simulink model "determine_attitude_quest"  (R2022a)
settings: Solver=VariableStepAuto  StartTime=0.0  StopTime=10.0  RelTol=1e-3
undefined symbols (not defined in the file or in its folder): IAU, km, s
libraries: aerolibutil x9, sharedtransform x3, vrlib x3, aerolibtransform2 x2, aerolibcelestial x1
settings Model: Creator=joshu  LastModifiedBy=joshu

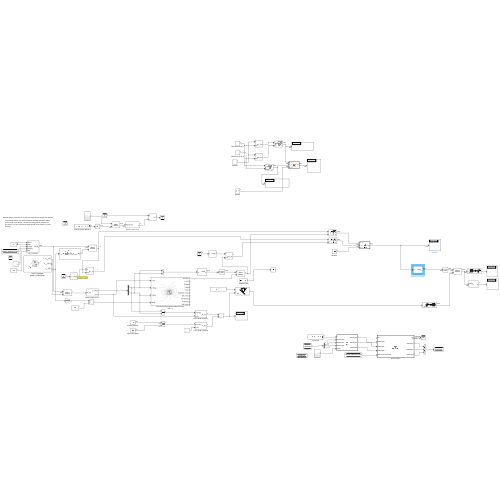
[thumbnail: Simulink's stored preview of the top-level diagram]
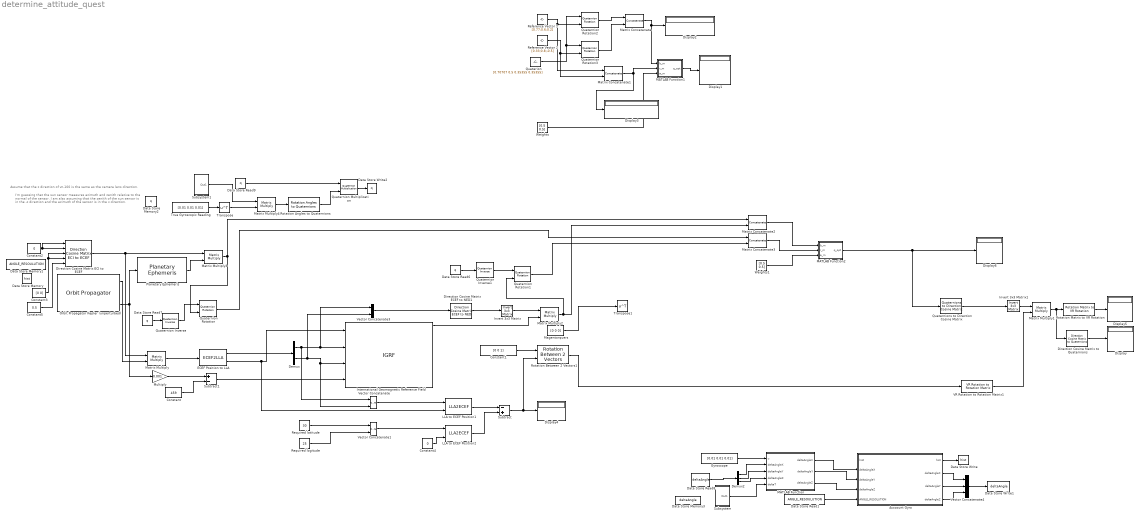
== system determine_attitude_quest ==
  note: I'm guessing that the sun sensor measures azimuth and zenith relative to the normal of the sensor. I am also assuming that the zenith of the sun sensor is in the -z direction and the azimuth of the sensor is in the x direction.
  note: Assume that the z direction of vn-100 is the same as the camera lens direction.
  Acccount Gyro : MATLAB Function  TreatAsAtomicUnit=on
  Constant : Constant  Value=459
  Constant1 : Constant  Value=[0 0 1]
  Constant2 : Constant  Value=0
  Constant3 : Constant  Value=[0 0]
  Constant4 : Constant  Value=0
  Constant5 : Constant  Value=0.5
  Data Store Memory : DataStoreMemory  DataStoreName=hist  WriteAfterWriteMsg=warning  InitialValue=1  ShowAdditionalParam=off  OutDataTypeStr=double  Dimensions=[100 100 100]
  Data Store Memory1 : DataStoreMemory  DataStoreName=ANGLE_RESOULUTION  WriteAfterWriteMsg=warning  InitialValue=100  ShowAdditionalParam=off
  Data Store Memory2 : DataStoreMemory  DataStoreName=q  WriteAfterWriteMsg=warning  InitialValue=[0.70707 0.5 0.35355 0.35355]  ShowAdditionalParam=off
  Data Store Memory3 : DataStoreMemory  DataStoreName=deltaAngle  WriteAfterWriteMsg=warning  InitialValue=[0 0 0]  ShowAdditionalParam=off
  Data Store Read1 : DataStoreRead  DataStoreName=ANGLE_RESOULUTION  IndexOptions=Index vector (dialog)  Indices=1  OutputSizes=1
  Data Store Read6 : DataStoreRead  DataStoreName=q  IndexOptions=Index vector (dialog)  Indices=1  OutputSizes=1
  Data Store Read7 : DataStoreRead  DataStoreName=q  IndexOptions=Index vector (dialog)  Indices=1  OutputSizes=1
  Data Store Read8 : DataStoreRead  DataStoreName=deltaAngle  IndexOptions=Index vector (dialog)  Indices=1  OutputSizes=1
  Data Store Read9 : DataStoreRead  DataStoreName=q  IndexOptions=Index vector (dialog)  Indices=1  OutputSizes=1
  Data Store Write : DataStoreWrite  DataStoreName=hist  IndexOptions=Index vector (dialog)  Indices=1  OutputSizes=1
  Data Store Write1 : DataStoreWrite  DataStoreName=deltaAngle  IndexOptions=Index vector (dialog)  Indices=1  OutputSizes=1
  Data Store Write2 : DataStoreWrite  DataStoreName=q  IndexOptions=Index vector (dialog)  Indices=1  OutputSizes=1
  Demux : Demux  Outputs=2
  Demux2 : Demux  Outputs=3
  Direction Cosine Matrix ECEF to NED1 : aerolibtransform2/Direction Cosine Matrix ECEF to NED
      settings: SourceProductBaseCode=AE
  Direction Cosine Matrix ECI to ECEF : aerolibtransform2/Direction Cosine Matrix ECI to ECEF  red=IAU-2000/2006  year=2013  month=January  day=1  hour=0  min=0  sec=0  deltaT=Day  errorflag=Error  extraparamflag=on
      settings: AttributesFormatString=%<red>  SourceProductBaseCode=AE
  Direction Cosine Matrix to Quaternions : sharedtransform/Direction Cosine Matrix  to Quaternions  aMode=0  action=None  tolerance=eps(2)
      settings: SourceProductBaseCode=AE,PW,DR,MT,VE
  Display{,1..6} (7 alike) : Display
  ECEF Position to LLA : ECEF2LLA
  Gyroscope : Constant  Value=[0.01 0.01 0.01]
  International Geomagnetic Reference Field : IGRF  month=January  day=1  year=2020  action=Warning
      settings: AttributesFormatString=%<generation>
  Invert 3x3 Matrix : aerolibutil/Invert  3x3 Matrix
  Invert 3x3 Matrix1 : aerolibutil/Invert  3x3 Matrix
  LLA to ECEF Position1 : LLA2ECEF
  LLA to ECEF Position2 : LLA2ECEF
  MATLAB Function : MATLAB Function  TreatAsAtomicUnit=on
  MATLAB Function1 : MATLAB Function  TreatAsAtomicUnit=on
  MATLAB Function2 : MATLAB Function  TreatAsAtomicUnit=on
  Magentorquers : Constant  Value=[0 0 0]
  Matrix Concatenate{,1..3} (4 alike) : Concatenate  Mode=Multidimensional array  ConcatenateDimension=2
  Matrix Multiply{,1..4} (5 alike) : Product  Multiplication=Matrix(*)
  Multiply : Gain  Gain=0.001
  Orbit Propagator Kepler (unperturbed) : OrbitPropagator  inertialPosition=[3649700.0 3308200.0 -4676600.0]  inertialVelocity=[-2750.8 6666.4 2573.4]  fixedPosition=[-4142689.0 -2676864.7 -4669861.6]  fixedVelocity=[1452.7 -6720.7 2568.1]  customR=3396200  customMu=4.305e13  customJ2=1.0826269e-03  customOmega=4.06125949e-3
  Planetary Ephemeris : aerolibcelestial/Planetary Ephemeris  kmflag=km,km/s  epochflag=Julian date  de=DE405  nCenter=Earth  nTarget=Sun  errorflag=Error  velflag=off
      settings: SourceProductBaseCode=AE
  Quaterion : Constant  Value=[0.70707 0.5 0.35355 0.35355]
  Quaternion Inverse : aerolibutil/Quaternion Inverse
  Quaternion Inverse1 : aerolibutil/Quaternion Inverse
  Quaternion Multiplication : aerolibutil/Quaternion Multiplication
  Quaternion Rotation{,1..3} (4 alike) : aerolibutil/Quaternion Rotation
  Quaternions to Direction Cosine Matrix : sharedtransform/Quaternions to  Direction Cosine Matrix  aMode=aMode
      settings: SourceProductBaseCode=AE,PW,DR,MT,VE
  Reference Vector 1 : Constant  Value=[0.77;0.6;0.2]
  Reference Vector 2 : Constant  Value=[0.33;0.8;-0.5]
  Required latitude : Constant  Value=30  VectorParams1D=off
  Required logitude : Constant  Value=25  VectorParams1D=off
  Rotation Angles to Quaternions : sharedtransform/Rotation Angles to Quaternions  rotationOrder=ZYX  aMode=aMode
      settings: SourceProductBaseCode=AE,PW,DR,MT,VE
  Rotation Between 2 Vectors1 : vrlib/Utilities/Rotation Between 2 Vectors
      settings: SourceProductBaseCode=SL
  Rotation Matrix to VR Rotation : vrlib/Utilities/Rotation Matrix to VR Rotation  maxzero=1e-12
      settings: SourceProductBaseCode=SL
  Subsystem : Subsystem
  Subsystem1 : Subsystem
  Subtract : Sum  Inputs=-+
  Subtract1 : Sum  Inputs=+-
  Transpose : Math  Operator=transpose
  Transpose1 : Math  Operator=transpose
  True Gyroscopic Reading : Constant  Value=[0.01 0.01 0.01]
  VR Rotation to Rotation Matrix1 : vrlib/Utilities/VR Rotation to Rotation Matrix  maxzero=1e-12
      settings: SourceProductBaseCode=SL
  Vector Concatenate : Concatenate
  Vector Concatenate1 : Concatenate
  Vector Concatenate3 : Concatenate
  Vector Concatenate4 : Concatenate  NumInputs=3
  Weights : Constant  Value=[0.5 0.5]
  Weights1 : Constant  Value=[0.5 0.5]
  wires:
  Quaternion Rotation1/1 -> Matrix Concatenate3/2
  Rotation Between 2 Vectors1/1 -> VR Rotation to Rotation Matrix1/1
  Subtract/1 -> Rotation Between 2 Vectors1/2, Display4/1
  MATLAB Function2/1(q_opt) -> Quaternions to Direction Cosine Matrix/1, Display6/1
  Data Store Read1/1 -> Acccount Gyro/5(ANGLE_RESOLUTION)
  Invert 3x3 Matrix1/1 -> Matrix Multiply1/1
  Direction Cosine Matrix ECEF to NED1/1 -> Invert 3x3 Matrix/1
  Acccount Gyro/1(hist) -> Data Store Write/1
  Subtract1/1 -> International Geomagnetic Reference Field/4
  Gyroscope/1 -> MATLAB Function/1(u)
  VR Rotation to Rotation Matrix1/1 -> Matrix Multiply1/2
  Vector Concatenate1/1 -> LLA to ECEF Position2/1
  Rotation Matrix to VR Rotation/1 -> Display5/1
  Vector Concatenate3/1 -> Direction Cosine Matrix ECEF to NED1/1
  Constant5/1 -> Direction Cosine Matrix ECI to ECEF/5
  Orbit Propagator Kepler (unperturbed)/1 -> Matrix Multiply/2
  Constant4/1 -> LLA to ECEF Position2/2
  Matrix Multiply2/1 -> Matrix Concatenate2/2, Quaternion Rotation1/2
  ECEF Position to LLA/1 -> Demux/1
  Constant2/1 -> Direction Cosine Matrix ECI to ECEF/2, Direction Cosine Matrix ECI to ECEF/1
  Direction Cosine Matrix to Quaternions/1 -> Display/1
  ECEF Position to LLA/2 -> LLA to ECEF Position1/2, International Geomagnetic Reference Field/1
  International Geomagnetic Reference Field/1 -> Matrix Multiply2/2
  Invert 3x3 Matrix/1 -> Matrix Multiply2/1
  Magentorquers/1 -> Transpose1/1
  LLA to ECEF Position1/1 -> Subtract/1
  Required logitude/1 -> Vector Concatenate1/2
  Direction Cosine Matrix ECI to ECEF/1 -> Matrix Multiply/1, Matrix Multiply3/1
  Required latitude/1 -> Vector Concatenate1/1
  Demux/2 -> Vector Concatenate/2, International Geomagnetic Reference Field/3, Vector Concatenate3/2
  Matrix Multiply/1 -> ECEF Position to LLA/1
  Matrix Multiply3/1 -> Matrix Concatenate2/1, Quaternion Rotation/2
  Planetary Ephemeris/1 -> Matrix Multiply3/2
  LLA to ECEF Position2/1 -> Subtract/2
  Vector Concatenate/1 -> LLA to ECEF Position1/1
  Multiply/1 -> Subtract1/1
  Quaternion Rotation/1 -> Matrix Concatenate3/1
  Constant1/1 -> Rotation Between 2 Vectors1/1
  Constant/1 -> Subtract1/2
  Demux/1 -> Vector Concatenate3/1, International Geomagnetic Reference Field/2, Vector Concatenate/1
  Matrix Multiply1/1 -> Rotation Matrix to VR Rotation/1, Direction Cosine Matrix to Quaternions/1
  Constant3/1 -> Direction Cosine Matrix ECI to ECEF/4, Direction Cosine Matrix ECI to ECEF/3
  Orbit Propagator Kepler (unperturbed)/3 -> Multiply/1, Planetary Ephemeris/1
  Quaternion Inverse/1 -> Quaternion Rotation/1
  Quaternion Inverse1/1 -> Quaternion Rotation1/1
  Data Store Read6/1 -> Quaternion Inverse1/1
  Data Store Read7/1 -> Quaternion Inverse/1
  Demux2/1 -> MATLAB Function/2("deltaAngleX ")
  Demux2/2 -> MATLAB Function/3("deltaAngleY ")
  Demux2/3 -> MATLAB Function/4("deltaAngleZ ")
  Subsystem/1(Out1) -> MATLAB Function/5(deltaT)
  MATLAB Function/1(deltaAngleX) -> Acccount Gyro/2("deltaAngleX ")
  MATLAB Function/2(deltaAngleY) -> Acccount Gyro/3("deltaAngleY ")
  MATLAB Function/3(deltaAngleZ) -> Acccount Gyro/4("deltaAngleZ ")
  Data Store Read8/1 -> Demux2/1
  Acccount Gyro/2(deltaAngleX) -> Vector Concatenate4/1
  Acccount Gyro/3(deltaAngleY) -> Vector Concatenate4/2
  Acccount Gyro/4(deltaAngleZ) -> Vector Concatenate4/3
  Vector Concatenate4/1 -> Data Store Write1/1
  True Gyroscopic Reading/1 -> Transpose/1
  Subsystem1/1(Out1) -> Matrix Multiply4/1
  Matrix Multiply4/1 -> Rotation Angles to Quaternions/1
  Data Store Read9/1 -> Quaternion Multiplication/1
  Rotation Angles to Quaternions/1 -> Quaternion Multiplication/2
  Quaternion Multiplication/1 -> Data Store Write2/1
  Transpose/1 -> Matrix Multiply4/2
  MATLAB Function1/1(q_opt) -> Display1/1
  Quaterion/1 -> Quaternion Rotation3/1, Quaternion Rotation2/1
  Reference Vector 2/1 -> Matrix Concatenate1/2, Quaternion Rotation3/2
  Reference Vector 1/1 -> Matrix Concatenate1/1, Quaternion Rotation2/2
  Quaternion Rotation2/1 -> Matrix Concatenate/1
  Quaternion Rotation3/1 -> Matrix Concatenate/2
  Weights/1 -> MATLAB Function1/3(a_m)
  Matrix Concatenate1/1 -> Display3/1, MATLAB Function1/2(r_m)
  Matrix Concatenate/1 -> Display2/1, MATLAB Function1/1(b_m)
  Matrix Concatenate2/1 -> MATLAB Function2/1(b_m)
  Matrix Concatenate3/1 -> MATLAB Function2/2(r_m)
  Weights1/1 -> MATLAB Function2/3(a_m)
  Quaternions to Direction Cosine Matrix/1 -> Invert 3x3 Matrix1/1

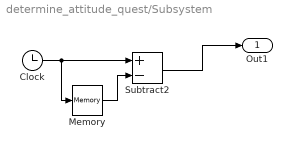
== system determine_attitude_quest/Subsystem ==
  Clock : Clock
  Memory : Memory
  Subtract2 : Sum  Inputs=+-
  Out1 : Outport
  wires:
  Memory/1 -> Subtract2/2
  Clock/1 -> Memory/1, Subtract2/1
  Subtract2/1 -> Out1/1

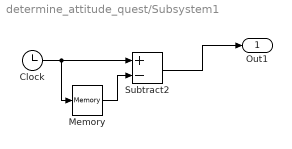
== system determine_attitude_quest/Subsystem1 ==
  Clock : Clock
  Memory : Memory
  Subtract2 : Sum  Inputs=+-
  Out1 : Outport
  wires:
  Memory/1 -> Subtract2/2
  Clock/1 -> Memory/1, Subtract2/1
  Subtract2/1 -> Out1/1

== matlab function determine_attitude_quest/Acccount Gyro ==
  data: hist input size=[100 100 100]; hist output; deltaAngleX input; deltaAngleY input; deltaAngleZ input; ANGLE_RESOLUTION input; deltaAngleX output; deltaAngleY output; deltaAngleZ output
function [hist,deltaAngleX,deltaAngleY,deltaAngleZ] = addMotion(hist,deltaAngleX,deltaAngleY,deltaAngleZ,ANGLE_RESOLUTION)
    %ANGLE_RESOLUTION = 500;

    if(deltaAngleX > 2*pi/ANGLE_RESOLUTION)
        hist = circshift(hist,1,1);
        deltaAngleX = deltaAngleX - 2*pi/ANGLE_RESOLUTION;
    end
    
    if(deltaAngleY > 2*pi/ANGLE_RESOLUTION)
        hist = circshift(hist,1,2);
        deltaAngleY = deltaAngleY - 2*pi/ANGLE_RESOLUTION;
    end
    
    if(deltaAngleZ > 2*pi/ANGLE_RESOLUTION)
        hist = circshift(hist,1,3);
        deltaAngleZ = deltaAngleZ - 2*pi/ANGLE_RESOLUTION;
    end

    if(deltaAngleX < -2*pi/ANGLE_RESOLUTION)
        hist = circshift(hist,1,100-1);
        deltaAngleX = deltaAngleX + 2*pi/ANGLE_RESOLUTION;
    end
    
    if(deltaAngleY < -2*pi/ANGLE_RESOLUTION)
        hist = circshift(hist,1,100-2);
        deltaAngleY = deltaAngleY + 2*pi/ANGLE_RESOLUTION;
    end
    
    if(deltaAngleZ < -2*pi/ANGLE_RESOLUTION)
        hist = circshift(hist,1,100-3);
        deltaAngleZ = deltaAngleZ + 2*pi/ANGLE_RESOLUTION;
    end
end

== matlab function determine_attitude_quest/MATLAB Function2 ==
  data: b_m input; q_opt output; r_m input; a_m input
function q_opt = quest(b_m, r_m, a_m)
  
v_b = b_m
v_i = r_m
w = a_m

[N,~] = size(w);

tolerance = 10e-5;


B = zeros(3);

for i = 1:N
B = B + a_m(i)*b_m(:,i)*r_m(:,i)'; %5.11
end

%B = (v_b.*repmat(w,[1,3])')*v_i'; % Eqn 38
Z = [B(2,3)-B(3,2); B(3,1)-B(1,3); B(1,2)-B(2,1)]; % Eqn 46
S = B + B'; % Eqn 45
sigma = trace(B); % Eqn 44

% Eqn 63
delta = det(S);
kappa = trace(delta*inv(S));

% Eqn 71
a = sigma^2 - kappa;
b = sigma^2 + Z'*Z;
c = delta + Z'*S*Z;
d = Z'*S^2*Z;
constant = a*b + c*sigma - d;

% Characteristic equation for Newton-Raphson method: (Eqn 70) 
%   f(lambda) = lambda^4 - (a + b)*lambda^2 - c*lambda + constant = 0
%   where, constant = a*b + c*sigma - d
lambda = sum(w); % Shuster1981 and markley1993
last_lambda = 0.0;
while abs(lambda - last_lambda) >= tolerance
    last_lambda = lambda;
    
    f = lambda^4 - (a + b)*lambda^2 - c*lambda + constant;
    f_dot = 4*lambda^3 - 2*(a + b)*lambda - c;
    lambda = lambda - f/f_dot;
end
  
% Eqn 66
omega = lambda;
alpha = omega^2 - sigma^2 + kappa;
beta  = omega - sigma;
gamma = (omega + sigma)*alpha - delta;

% Determine optimal quaternion
X = (alpha*eye(3) + beta*S + S^2)*Z; % Eqn 68
q_opt = [gamma; X]./sqrt(gamma^2 + norm(X)^2); % Eqn 69


end

== matlab function determine_attitude_quest/MATLAB Function ==
  data: u input; deltaAngleX output; deltaAngleX input; deltaAngleY input; deltaAngleZ input; deltaAngleY output; deltaAngleZ output; deltaT input
function [deltaAngleX,deltaAngleY,deltaAngleZ] = fcn(u,deltaAngleX,deltaAngleY,deltaAngleZ,deltaT)

deltaAngleX = deltaAngleX + u(1)*deltaT;
deltaAngleY = deltaAngleY + u(2)*deltaT;
deltaAngleZ = deltaAngleZ + u(3)*deltaT;

== matlab function determine_attitude_quest/MATLAB Function1 ==
  data: b_m input; q_opt output; r_m input; a_m input
function q_opt = quest(b_m, r_m, a_m)
  
v_b = b_m
v_i = r_m
w = a_m

[N,~] = size(w);

tolerance = 10e-5;


B = zeros(3);

for i = 1:N
B = B + a_m(i)*b_m(:,i)*r_m(:,i)'; %5.11
end

%B = (v_b.*repmat(w,[1,3])')*v_i'; % Eqn 38
Z = [B(2,3)-B(3,2); B(3,1)-B(1,3); B(1,2)-B(2,1)]; % Eqn 46
S = B + B'; % Eqn 45
sigma = trace(B); % Eqn 44

% Eqn 63
delta = det(S);
kappa = trace(delta*inv(S));

% Eqn 71
a = sigma^2 - kappa;
b = sigma^2 + Z'*Z;
c = delta + Z'*S*Z;
d = Z'*S^2*Z;
constant = a*b + c*sigma - d;

% Characteristic equation for Newton-Raphson method: (Eqn 70) 
%   f(lambda) = lambda^4 - (a + b)*lambda^2 - c*lambda + constant = 0
%   where, constant = a*b + c*sigma - d
lambda = sum(w); % Shuster1981 and markley1993
last_lambda = 0.0;
while abs(lambda - last_lambda) >= tolerance
    last_lambda = lambda;
    
    f = lambda^4 - (a + b)*lambda^2 - c*lambda + constant;
    f_dot = 4*lambda^3 - 2*(a + b)*lambda - c;
    lambda = lambda - f/f_dot;
end
  
% Eqn 66
omega = lambda;
alpha = omega^2 - sigma^2 + kappa;
beta  = omega - sigma;
gamma = (omega + sigma)*alpha - delta;

% Determine optimal quaternion
X = (alpha*eye(3) + beta*S + S^2)*Z; % Eqn 68
q_opt = [gamma; X]./sqrt(gamma^2 + norm(X)^2); % Eqn 69


end
